simulink model "AM"  (R2020b)
settings: Solver=VariableStepAuto  StartTime=0.0  StopTime=10.0  RelTol=1e-3  EnableMultiTasking=on
libraries: dsparch4 x2, simulink x1
settings Model: Creator=xiao'xin  LastModifiedBy=xiao'xin
settings DataIOCC: LimitDataPoints=on  ReturnWorkspaceOutputs=off
settings OptimizationCC: LifeSpan=inf
settings DebuggingCC: AllowSymbolicDim=off  SFUnexpectedBacktrackingDiag=warning  SFNoUnconditionalDefaultTransitionDiag=warning  SFExecutionAtInitializationDiag=none  ArithmeticOperatorsInVariantConditions=warning
settings ModelReferenceCC: PropagateSignalLabelsOutOfModel=off
settings SFSimCC: SimUseLocalCustomCode=off  CustomCodeUndefinedFunction=UseInterfaceOnly
settings RTWCC: RTWUseLocalCustomCode=off
settings CodeAppCC: StateflowObjectComments=on
settings GRTTargetCC: TargetLangStandard=C89/C90 (ANSI)
settings ConfigComp: CovMetricSettings=dw  CovSaveCumulativeToWorkspaceVar=on  CovSaveSingleToWorkspaceVar=on  CovExternalEMLEnable=off

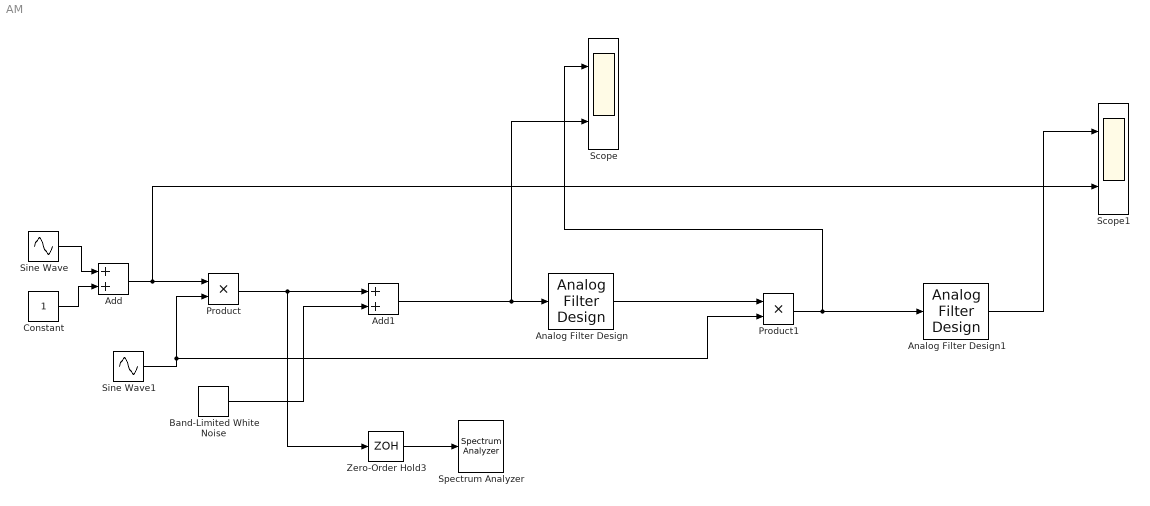
== system AM ==
  Add : Sum
  Add1 : Sum
  Analog Filter Design : dsparch4/Analog Filter Design  method=Butterworth  filttype=Bandpass  N=8  Wlo=9500*2*pi  Whi=10500*2*pi  Rp=2  Rs=40
  Analog Filter Design1 : dsparch4/Analog Filter Design  method=Butterworth  filttype=Lowpass  N=8  Wlo=1000*2*pi  Whi=10500*2*pi  Rp=2  Rs=40
  Band-Limited White Noise : simulink/Sources/Band-Limited White Noise  Cov=[0.01]  Ts=0.1  seed=[23341]
  Constant : Constant
  Product : Product
  Product1 : Product
  Scope : Scope  NumInputPorts=2
  Scope1 : Scope  NumInputPorts=2
  Sine Wave : Sin  Frequency=300*2*pi  SampleTime=0
  Sine Wave1 : Sin  Amplitude=5  Frequency=10000*2*pi  SampleTime=0
  Spectrum Analyzer : SpectrumAnalyzer
  Zero-Order Hold3 : ZeroOrderHold  SampleTime=0.00001
  wires:
  Sine Wave/1 -> Add/1
  Constant/1 -> Add/2
  Add/1 -> Scope1/2, Product/1
  Sine Wave1/1 -> Product1/2, Product/2
  Product/1 -> Zero-Order Hold3/1, Add1/1
  Add1/1 -> Scope/2, Analog Filter Design/1
  Analog Filter Design/1 -> Product1/1
  Product1/1 -> Analog Filter Design1/1, Scope/1
  Analog Filter Design1/1 -> Scope1/1
  Band-Limited White Noise/1 -> Add1/2
  Zero-Order Hold3/1 -> Spectrum Analyzer/1
